simulink library "CTRL_SPECCTRL_FB_STRAT1_SLAWHL"  (R2024b)
settings: Solver=VariableStepAuto  StartTime=0.0  StopTime=10.0  RelTol=1e-3
libraries: VUT_lib x1
settings Model: Creator=blatak  LastModifiedBy=blatak

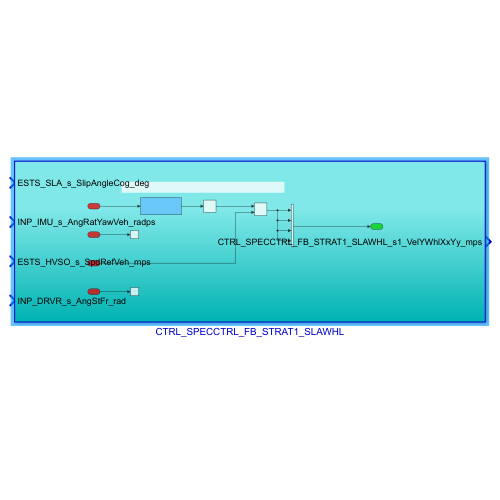
[thumbnail: Simulink's stored preview of the top-level diagram]
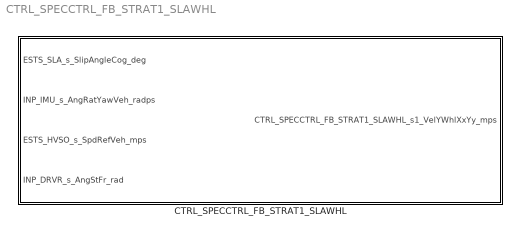
== system CTRL_SPECCTRL_FB_STRAT1_SLAWHL ==
  CTRL_SPECCTRL_FB_STRAT1_SLAWHL : Subsystem

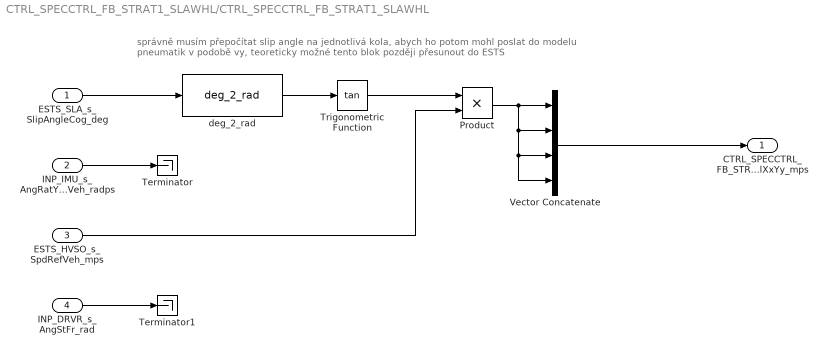
== system CTRL_SPECCTRL_FB_STRAT1_SLAWHL/CTRL_SPECCTRL_FB_STRAT1_SLAWHL ==
  note: správně musím přepočítat slip angle na jednotlivá kola, abych ho potom mohl poslat do modelu pneumatik v podobě vy, teoreticky možné tento blok později přesunout do ESTS
  ESTS_SLA_s_SlipAngleCog_deg : Inport
  INP_IMU_s_AngRatYawVeh_radps : Inport  Port=2
  ESTS_HVSO_s_SpdRefVeh_mps : Inport  Port=3
  INP_DRVR_s_AngStFr_rad : Inport  Port=4
  Product : Product
  Terminator : Terminator
  Terminator1 : Terminator
  Trigonometric Function : Trigonometry  Operator=tan
  Vector Concatenate : Concatenate  NumInputs=4  Mode=Multidimensional array
  deg_2_rad : VUT_lib/deg_2_rad  SystemSampleTime=-1  VariantActivationTime=update diagram  AllowFlexibleInterface=on  Latency=0  AutoFrameSizeCalculation=off
  CTRL_SPECCTRL_FB_STRAT1_SLAWHL_s1_VelYWhlXxYy_mps : Outport
  wires:
  INP_IMU_s_AngRatYawVeh_radps/1 -> Terminator/1
  Product/1 -> Vector Concatenate/4, Vector Concatenate/3, Vector Concatenate/2, Vector Concatenate/1
  ESTS_SLA_s_SlipAngleCog_deg/1 -> deg_2_rad/1
  Trigonometric Function/1 -> Product/1
  Vector Concatenate/1 -> CTRL_SPECCTRL_FB_STRAT1_SLAWHL_s1_VelYWhlXxYy_mps/1
  INP_DRVR_s_AngStFr_rad/1 -> Terminator1/1
  ESTS_HVSO_s_SpdRefVeh_mps/1 -> Product/2
  deg_2_rad/1 -> Trigonometric Function/1
